simulink model "NMRAC_MIMO_SIM"  (R2024a)
settings: Solver=VariableStepAuto  StartTime=0.0  StopTime=Tsim  MaxStep=Ts  RelTol=1e-3
values from neighbouring files (symbols this model uses):
  A = Am    [NMRAC_SIM.m]
  a = 1    [NMRAC_SIM.m]
  Am = [0 1; 0 -0.1]    [NMRAC_SIM.m]
  B = Bm    [NMRAC_SIM.m]
  Bm = [1 0; 0 1]    [NMRAC_SIM.m]
  lambda = 0.01.*[1 0; 0 1]    [NMRAC_SIM.m]
  P = [1 0; 0 1]    [NMRAC_SIM.m]
  theta = theta + dtheta * Ts    [NMRAC_SIM.m]
  theta_m = [1 1; 1 1]    [NMRAC_SIM.m]
undefined symbols (not defined in the file or in its folder): x0, x_r, xm0
settings Model: Creator=dalimwahby  LastModifiedBy=dalimwahby

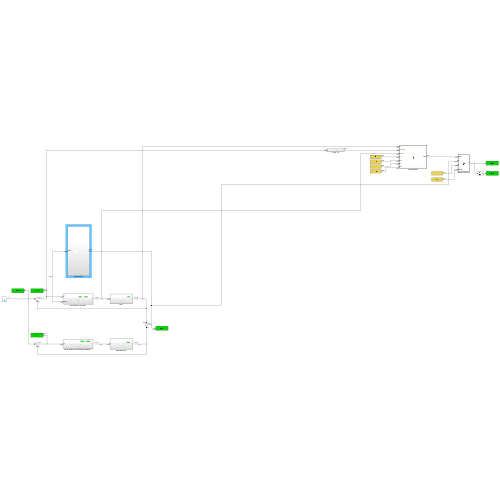
[thumbnail: Simulink's stored preview of the top-level diagram]
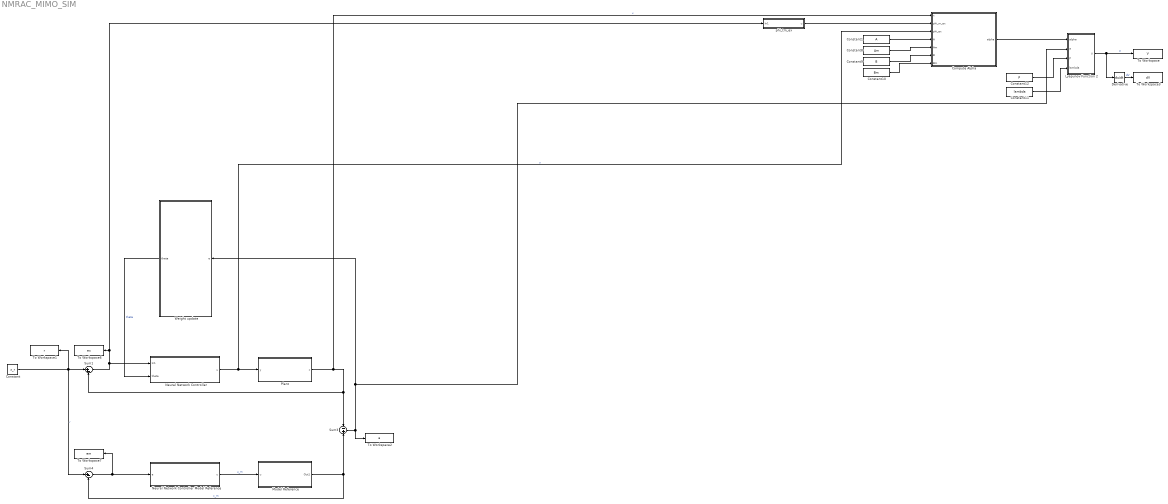
== system NMRAC_MIMO_SIM ==
  Compute Alpha : MATLAB Function  TreatAsAtomicUnit=on
  Constant : Constant  Value=x_r
  Constant1 : Constant  Value=A
  Constant10 : Constant  Value=Bm
  Constant11 : Constant  Value=lambda
  Constant12 : Constant  Value=P
  Constant8 : Constant  Value=Am
  Constant9 : Constant  Value=B
  Derivative : Derivative
  Lyapunov Function 2 : MATLAB Function  TreatAsAtomicUnit=on
  Model Reference : Subsystem
  Neural Network Controller : Subsystem
  "Neural Network Controller Model Reference " : Subsystem
  Plant : Subsystem
  Sum1 : Sum  Inputs=|+-
  Sum3 : Sum  Inputs=-+
  Sum4 : Sum  Inputs=|+-
  To Workspace : ToWorkspace  VariableName=V  SaveFormat=Timeseries  SampleTime=-1
  To Workspace1 : ToWorkspace  VariableName=r  SaveFormat=Timeseries  SampleTime=-1
  To Workspace2 : ToWorkspace  VariableName=e  SaveFormat=Timeseries  SampleTime=-1
  To Workspace3 : ToWorkspace  VariableName=dV  SaveFormat=Timeseries  SampleTime=-1
  To Workspace6 : ToWorkspace  VariableName=ex  SaveFormat=Timeseries  SampleTime=-1
  To Workspace7 : ToWorkspace  VariableName=em  SaveFormat=Timeseries  SampleTime=-1
  Weight update : Subsystem
  phi_tm_ex : Subsystem
  wires:
  Plant/1(x) -> Compute Alpha/1(x), Sum3/1, Sum1/2  "x"
  Constant/1 -> Sum4/1, To Workspace1/1, Sum1/1  "r"
  Model Reference/1(Out1) -> Sum4/2, Sum3/2  "x_m"
  Sum4/1 -> "Neural Network Controller Model Reference "/1(e), To Workspace7/1
  Sum1/1 -> phi_tm_ex/1(In1), To Workspace6/1, Neural Network Controller/1(In1)
  Neural Network Controller/1(u) -> Compute Alpha/3(phi_ex), Plant/1(y)  "u"
  "Neural Network Controller Model Reference "/1(u) -> Model Reference/1(u)  "u_m"
  phi_tm_ex/1(u) -> Compute Alpha/2(phi_m_ex)
  Sum3/1 -> Lyapunov Function 2/2(e), Weight update/1(e), To Workspace2/1
  Weight update/1(theta) -> Neural Network Controller/2(theta)  "theta"
  Compute Alpha/1(alpha) -> Lyapunov Function 2/1(alpha)
  Lyapunov Function 2/1(V) -> Derivative/1, To Workspace/1  "V"
  Constant1/1 -> Compute Alpha/4(A)
  Constant8/1 -> Compute Alpha/5(Am)
  Constant9/1 -> Compute Alpha/6(B)
  Constant10/1 -> Compute Alpha/7(Bm)
  Constant11/1 -> Lyapunov Function 2/4(lambda)
  Constant12/1 -> Lyapunov Function 2/3(P)
  Derivative/1 -> To Workspace3/1  "dV"

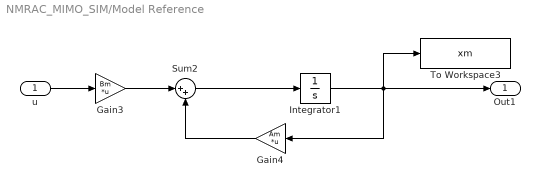
== system NMRAC_MIMO_SIM/Model Reference ==
  u : Inport
  Gain3 : Gain  Gain=Bm  Multiplication=Matrix(K*u)
  Gain4 : Gain  Gain=Am  Multiplication=Matrix(K*u)
  Integrator1 : Integrator  InitialCondition=xm0
  Sum2 : Sum  Inputs=|++
  To Workspace3 : ToWorkspace  VariableName=xm  SaveFormat=Timeseries  SampleTime=-1
  Out1 : Outport
  wires:
  u/1 -> Gain3/1
  Gain3/1 -> Sum2/1
  Sum2/1 -> Integrator1/1
  Gain4/1 -> Sum2/2
  Integrator1/1 -> Out1/1, To Workspace3/1, Gain4/1

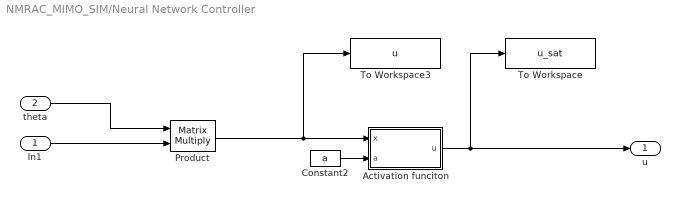
== system NMRAC_MIMO_SIM/Neural Network Controller ==
  In1 : Inport
  theta : Inport  Port=2
  Activation funciton : MATLAB Function  TreatAsAtomicUnit=on
  Constant2 : Constant  Value=a
  Product : Product  Multiplication=Matrix(*)
  To Workspace : ToWorkspace  VariableName=u_sat  SaveFormat=Timeseries  SampleTime=-1
  To Workspace3 : ToWorkspace  VariableName=u  SaveFormat=Timeseries  SampleTime=-1
  u : Outport
  wires:
  Activation funciton/1(u) -> To Workspace/1, u/1
  Product/1 -> To Workspace3/1, Activation funciton/1(x)
  In1/1 -> Product/2
  Constant2/1 -> Activation funciton/2(a)
  theta/1 -> Product/1

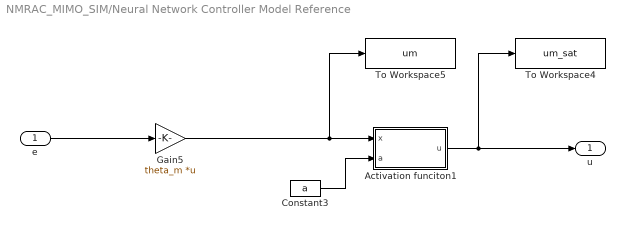
== system NMRAC_MIMO_SIM/Neural Network Controller Model Reference  ==
  e : Inport
  Activation funciton1 : MATLAB Function  TreatAsAtomicUnit=on
  Constant3 : Constant  Value=a
  Gain5 : Gain  Gain=theta_m  Multiplication=Matrix(K*u)
  To Workspace4 : ToWorkspace  VariableName=um_sat  SaveFormat=Timeseries  SampleTime=-1
  To Workspace5 : ToWorkspace  VariableName=um  SaveFormat=Timeseries  SampleTime=-1
  u : Outport
  wires:
  e/1 -> Gain5/1
  Activation funciton1/1(u) -> u/1, To Workspace4/1
  Gain5/1 -> To Workspace5/1, Activation funciton1/1(x)
  Constant3/1 -> Activation funciton1/2(a)

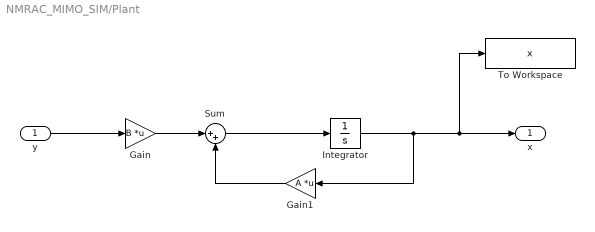
== system NMRAC_MIMO_SIM/Plant ==
  y : Inport
  Gain : Gain  Gain=B  Multiplication=Matrix(K*u)
  Gain1 : Gain  Gain=A  Multiplication=Matrix(K*u)
  Integrator : Integrator  InitialCondition=x0
  Sum : Sum  Inputs=|++
  To Workspace : ToWorkspace  VariableName=x  SaveFormat=Timeseries  SampleTime=-1
  x : Outport
  wires:
  y/1 -> Gain/1
  Sum/1 -> Integrator/1
  Integrator/1 -> Gain1/1, x/1, To Workspace/1
  Gain/1 -> Sum/1
  Gain1/1 -> Sum/2

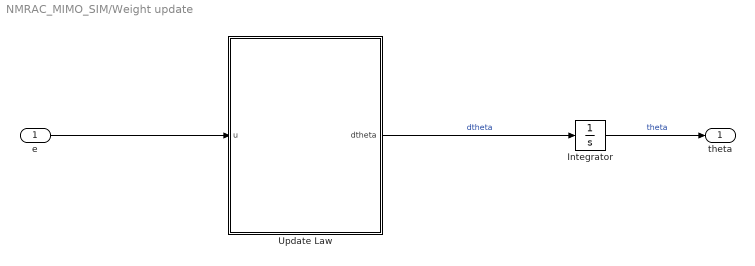
== system NMRAC_MIMO_SIM/Weight update ==
  e : Inport
  Integrator : Integrator  InitialCondition=theta
  Update Law : MATLAB Function  TreatAsAtomicUnit=on
  theta : Outport
  wires:
  Integrator/1 -> theta/1  "theta"
  Update Law/1(dtheta) -> Integrator/1  "dtheta"
  e/1 -> Update Law/1(u)

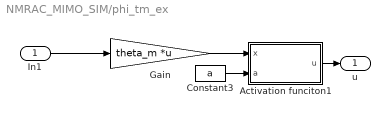
== system NMRAC_MIMO_SIM/phi_tm_ex ==
  In1 : Inport
  Activation funciton1 : MATLAB Function  TreatAsAtomicUnit=on
  Constant3 : Constant  Value=a
  Gain : Gain  Gain=theta_m  Multiplication=Matrix(K*u)
  u : Outport
  wires:
  Gain/1 -> Activation funciton1/1(x)
  In1/1 -> Gain/1
  Activation funciton1/1(u) -> u/1
  Constant3/1 -> Activation funciton1/2(a)

== matlab function NMRAC_MIMO_SIM/Neural Network Controller Model Reference /Activation funciton1 ==
  data: x input; u output; a input
function u = sigmoid(x, a)

u = 2.*(1-exp(-a.*x))./(a.*(1+exp(-a.*x)));

== matlab function NMRAC_MIMO_SIM/Neural Network Controller/Activation funciton ==
  data: x input; u output; a input
function  u = sigmoid(x, a)

u = 2.*(1-exp(-a.*x))./(a.*(1+exp(-a.*x)));

== matlab function NMRAC_MIMO_SIM/Weight update/Update Law ==
  data: u input; dtheta output
function dtheta = fcn(u)


SIGMA_plus = inv((B*dsigma_ex)'*B*dsigma_ex)*(B*dsigma_ex)'; % Pseudo inverse
ex_plus = ex'*inv(ex'*ex);

dtheta = [0.1 0.1; 0.1 0.1];
% dtheta = [0 0; 0 0];

== matlab function NMRAC_MIMO_SIM/phi_tm_ex/Activation funciton1 ==
  data: x input; u output; a input
function u = sigmoid(x, a)

u = 2.*(1-exp(-a.*x))./(a.*(1+exp(-a.*x)));

== matlab function NMRAC_MIMO_SIM/Lyapunov Function 2 ==
  data: alpha input; e input; V output; P input; lambda input
function V = fcn(alpha, e, P, lambda)

V = e'*P*e + alpha'*inv(lambda)*alpha;

== matlab function NMRAC_MIMO_SIM/Compute Alpha ==
  data: x input; alpha output; phi_m_ex input; phi_ex input; A input; Am input; B input; Bm input
function alpha = fcn(x, phi_m_ex, phi_ex, A, Am, B, Bm)

alpha = (Am-A)*x + Bm*phi_m_ex - B*phi_ex;
